simulink model "task2e"  (R2019b)
settings: Solver=ode45  StartTime=0.0  StopTime=10.0  RelTol=1e-3
values from neighbouring files (symbols this model uses):
  g = 9.8    [task1.m]    (also in task2c.m; task2e.m = 9.81; task2f.m = 9.81)
  l = l_hat_linf    [task1.m]    (also in task2c.m = 0.3; task2e.m = 0.3; task2f.m = 0.3)
  V = linf.V    [task2e.m]    (also in task2f.m)
undefined symbols (not defined in the file or in its folder): k1, ms, mw
settings Model: Creator=NicSch02  LastModifiedBy=NicSch02
settings OptimizationCC: LifeSpan=inf
settings DebuggingCC: SFExecutionAtInitializationDiag=none  ArithmeticOperatorsInVariantConditions=warning
settings HardwareCC: ProdBitPerSizeT=32  ProdBitPerPtrDiffT=32  ProdWordSize=32  ProdHWDeviceType=Specified
settings SFSimCC: CustomCodeUndefinedFunction=UseInterfaceOnly
settings CodeAppCC: StateflowObjectComments=on

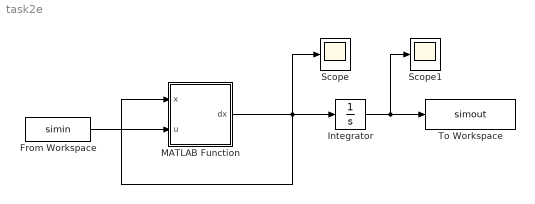
== system task2e ==
  From Workspace : FromWorkspace  VariableName=simin  SampleTime=0
  Integrator : Integrator
  MATLAB Function : MATLAB Function  TreatAsAtomicUnit=on
  Scope : Scope
  Scope1 : Scope
  To Workspace : ToWorkspace  VariableName=simout  SaveFormat=Timeseries  SampleTime=-1
  wires:
  MATLAB Function/1(dx) -> Scope/1, MATLAB Function/1(x), Integrator/1
  Integrator/1 -> Scope1/1, To Workspace/1
  From Workspace/1 -> MATLAB Function/2(u)

== matlab function task2e/MATLAB Function ==
  data: x input; g parameter; dx output; l parameter; u input; ms parameter; mw parameter; V parameter; k1 parameter
function dx = fcn(x,g,l,u, ms, mw, V, k1)
dx = [0;0;0;0];

dx(1) = x(3);
dx(2) = x(4);
dx(3) = (1/(mw+ms(1-cos(x(2))^2)))*(V*u - k1*x(3) + ms*l*x(4)^2*sin(x(2)) - ms*g*sin(x(2))*cos(x(2)));
dx(4) = (1/(1-(ms/(mw+ms))*cos(x(2))^2))*(g*sin(x(2)) - (cos(x(2))/(mw+ms))*(V*u-k1*x(3)) - ((ms/(mw+ms))*l*x(4)^2)*sin(x(2))*cos(x(2)));
